simulink model "task_3s"  (R2021a)
settings: Solver=VariableStepAuto  StartTime=0  StopTime=140  RelTol=1e-3
values from neighbouring files (symbols this model uses):
  a0 = 600    [task_2.m]    (also in task_3.m)
  a1 = 4e3    (= 4000)    [task_2.m]    (also in task_3.m)
  a2 = 7.2e3    (= 7200)    [task_2.m]    (also in task_3.m)
  A_line = pi*D_line^2/4    (= 0.502654824574)    [task_2.m]    (also in task_3.m)
  A_p = pi*D_p^2/4    (= 0.441786466911)    [task_2.m]    (also in task_3.m)
  A_tank = pi*D_tank^2/4    (= 28.2743338823)    [task_2.m]    (also in task_3.m)
  beta_3 = 78*pi/180    (= 1.36135681656)    [task_2.m]    (also in task_3.m)
  Cd = 0.9    [task_2.m]    (also in task_3.m)
  D_line = 0.8    [task_2.m]    (also in task_3.m)
  D_p = 0.75    [task_2.m]    (also in task_3.m)
  D_w = 3.5    [task_2.m]    (also in task_3.m)
  g = 9.81    [task_2.m]    (also in task_3.m)
  h0 = 10    [task_2.m]    (also in task_3.m)
  h2 = 175    [task_2.m]    (also in task_3.m)
  h_tank_0 = 7.47    [task_2.m]    (also in task_3.m)
  J = 4.6e5    (= 460000)    [task_2.m]    (also in task_3.m)
  K = 2e9    (= 2000000000)    [task_2.m]    (also in task_3.m)
  L_line = 5    [task_2.m]    (also in task_3.m)
  L_p = 220    [task_2.m]    (also in task_3.m)
  lambda = 5e-3    (= 0.005)    [task_2.m]    (also in task_3.m)
  lambda_p = 1e-4    (= 0.0001)    [task_2.m]    (also in task_3.m)
  omega_t = 15    [task_2.m]    (also in task_3.m)
  p_amb = 1e5    (= 100000)    [task_2.m]    (also in task_3.m)
  psi = 0.97    [task_2.m]    (also in task_3.m)
  rho = 1000    [task_2.m]    (also in task_3.m)
  Rv = (Av0/pi)^(1/2)    (= 0.398942280401)    [task_2.m]    (also in task_3.m)
  V_c = 0.27    [task_2.m]    (also in task_3.m)
  V_p = A_p*L_p    (= 97.1930227204)    [task_2.m]    (also in task_3.m)
  x_v = 0.5    [task_2.m]    (also in task_3.m)
undefined symbols (not defined in the file or in its folder): magnitude
settings Model: Creator=Jihai  LastModifiedBy=Shinya
settings SolverCC: AlgebraicLoopSolver=TrustRegion
settings OptimizationCC: BlockReduction=off  DefaultParameterBehavior=Inlined  BufferReuse=off
settings DebuggingCC: SFMachineParentedDataDiag=warning

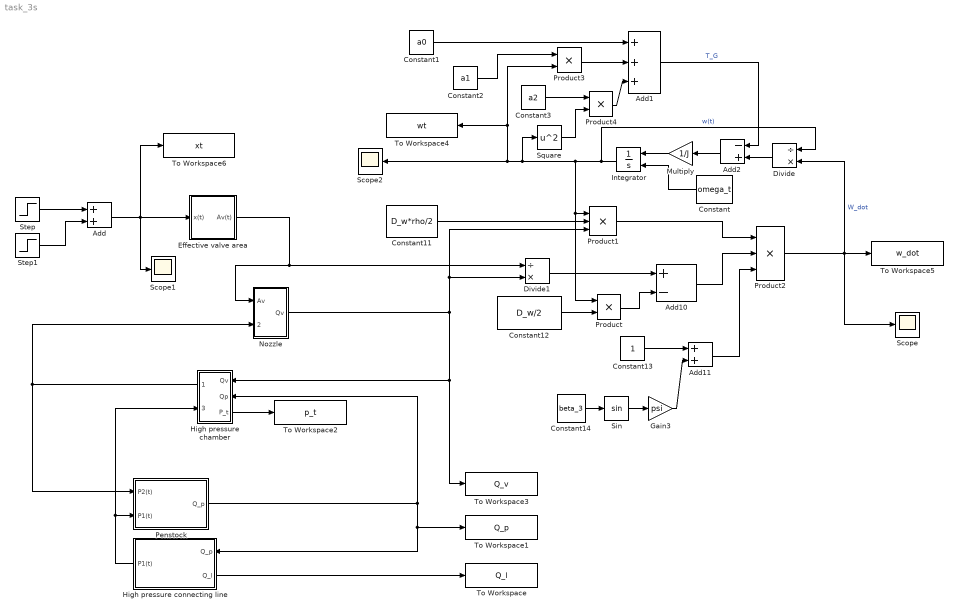
== system task_3s ==
  Add : Sum
  Add1 : Sum  Inputs=+++
  Add10 : Sum  Inputs=+-
  Add11 : Sum
  Add2 : Sum  Inputs=-+
  Constant : Constant  Value=omega_t
  Constant1 : Constant  Value=a0
  Constant11 : Constant  Value=D_w*rho/2
  Constant12 : Constant  Value=D_w/2
  Constant13 : Constant
  Constant14 : Constant  Value=beta_3
  Constant2 : Constant  Value=a1
  Constant3 : Constant  Value=a2
  Divide : Product  Inputs=/*
  Divide1 : Product  Inputs=/*
  Effective valve area : Subsystem
  Gain3 : Gain  Gain=psi
  High pressure chamber : Subsystem
      settings: PortSchema="{\"entries\":[{\"content\":{\"sides\":[{\"content\":{\"connectorIds\":[\"In1\",\"In2\",\"Out2\"]},\"type\":\"ConnectorPlacement.EquallySpacedRectSide\",\"uuid\":\"294ea827-fdb7-421d-abcf-acc1f7a75503\"},{\"content\":{\"connectorIds\":[\"Out1\",\"In3\"],\"side\":\"RIGHT\"},\"type\":\"ConnectorPlacement.EquallySpacedRectSide\",\"uuid\":\"1a834a5b-f580-4f55-8c0d-9c69e06391e8\"},{\"content\":{\"connectorIds\":[],\"side\":\"TOP\"},\"type\":\"ConnectorPlacement.EquallySpacedRectSide\",\"uuid\":\"b81bcc01-80a0-4387-ac31-2fde5e1e9cb3\"}]},\"type\":\"ConnectorPlacement.EquallySpacedConnector\",\"uuid\":\"9662d0fd-ac37-41a3-b53f-5a17ebe7bc5c\"}],\"packageUris\":[\"http://schema.mathworks.com/mf0/Connector/R2020b\"],\"version\":\"1.0\"}"
  High pressure connecting line : Subsystem
      settings: PortSchema="{\"entries\":[{\"content\":{\"sides\":[{\"content\":{\"connectorIds\":[\"In1\",\"Out2\"]},\"type\":\"ConnectorPlacement.EquallySpacedRectSide\",\"uuid\":\"6ad556de-4b40-4685-9767-8ac44a5f7b94\"},{\"content\":{\"connectorIds\":[\"Out1\"],\"side\":\"RIGHT\"},\"type\":\"ConnectorPlacement.EquallySpacedRectSide\",\"uuid\":\"0688f997-fb3f-4a41-bc89-421b9c81a19d\"},{\"content\":{\"connectorIds\":[],\"side\":\"TOP\"},\"type\":\"ConnectorPlacement.EquallySpacedRectSide\",\"uuid\":\"6829f08e-af19-4bca-bd06-6859c9ab2125\"}]},\"type\":\"ConnectorPlacement.EquallySpacedConnector\",\"uuid\":\"be56aa87-e3b2-4709-bfeb-a635322ac678\"}],\"packageUris\":[\"http://schema.mathworks.com/mf0/Connector/R2020b\"],\"version\":\"1.0\"}"
  Integrator : Integrator  InitialConditionSource=external
  Multiply : Gain  Gain=1/J
  Nozzle : Subsystem
  Penstock : Subsystem
  Product : Product
  Product1 : Product  Inputs=3
  Product2 : Product  Inputs=3
  Product3 : Product
  Product4 : Product
  Scope : Scope
  Scope1 : Scope
  Scope2 : Scope
  Sin : Trigonometry
  Square : Math  Operator=square  SaturateOnIntegerOverflow=on
  Step : Step  Time=20  Before=x_v  After=0.8  SampleTime=0
  Step1 : Step  Time=100  After=-0.7  SampleTime=0
  To Workspace : ToWorkspace  VariableName=Q_l  SampleTime=-1
  To Workspace1 : ToWorkspace  VariableName=Q_p  SampleTime=-1
  To Workspace2 : ToWorkspace  VariableName=p_t  SampleTime=-1
  To Workspace3 : ToWorkspace  VariableName=Q_v  SampleTime=-1
  To Workspace4 : ToWorkspace  VariableName=wt  SaveFormat=Timeseries  SampleTime=-1
  To Workspace5 : ToWorkspace  VariableName=w_dot  SaveFormat=Timeseries  SampleTime=-1
  To Workspace6 : ToWorkspace  VariableName=xt  SaveFormat=Timeseries  SampleTime=-1
  wires:
  High pressure chamber/1(P2(t)) -> Penstock/1(P2(t)), Nozzle/2(P2(t))
  Constant11/1 -> Product1/2
  Divide1/1 -> Add10/1
  Product1/1 -> Product2/1
  Add10/1 -> Product2/2
  Constant13/1 -> Add11/1
  Constant14/1 -> Sin/1
  Sin/1 -> Gain3/1
  Gain3/1 -> Add11/2
  Add11/1 -> Product2/3
  Product2/1 -> Divide/2, To Workspace5/1, Scope/1  "W_dot"
  High pressure connecting line/1(P1(t)) -> High pressure chamber/3(P1(t)), Penstock/2(P1(t))
  High pressure connecting line/2(Q_l) -> To Workspace/1
  Penstock/1(Q_p) -> High pressure chamber/2(Qp), High pressure connecting line/1(Q_p), To Workspace1/1
  Effective valve area/1(Av(t)) -> Nozzle/1(Av), Divide1/1
  High pressure chamber/2(P_t) -> To Workspace2/1
  Add/1 -> Scope1/1, To Workspace6/1, Effective valve area/1(x(t))
  Step/1 -> Add/1
  Step1/1 -> Add/2
  Nozzle/1(Qv) -> Product1/3, Divide1/2, To Workspace3/1, High pressure chamber/1(Qv)
  Constant/1 -> Integrator/2
  Product/1 -> Add10/2
  Constant12/1 -> Product/2
  Integrator/1 -> Divide/1, Square/1, To Workspace4/1, Product3/2, Scope2/1, Product1/1, Product/1  "w(t)"
  Divide/1 -> Add2/2
  Add1/1 -> Add2/1  "T_G"
  Add2/1 -> Multiply/1
  Multiply/1 -> Integrator/1
  Constant1/1 -> Add1/1
  Constant2/1 -> Product3/1
  Product4/1 -> Add1/3
  Product3/1 -> Add1/2
  Constant3/1 -> Product4/1
  Square/1 -> Product4/2

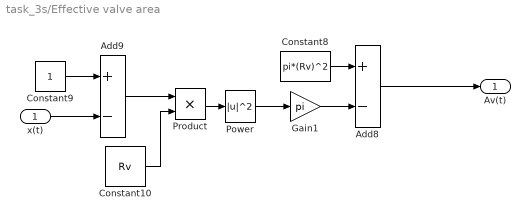
== system task_3s/Effective valve area ==
  x(t) : Inport
  Add8 : Sum  Inputs=+-
  Add9 : Sum  Inputs=+-
  Constant10 : Constant  Value=Rv
  Constant8 : Constant  Value=pi*(Rv)^2
  Constant9 : Constant
  Gain1 : Gain  Gain=pi
  Power : Math  Operator=magnitude^2  SaturateOnIntegerOverflow=on
  Product : Product
  Av(t) : Outport
  wires:
  Constant8/1 -> Add8/1
  Constant10/1 -> Product/2
  Add8/1 -> Av(t)/1
  Constant9/1 -> Add9/1
  Gain1/1 -> Add8/2
  Add9/1 -> Product/1
  Product/1 -> Power/1
  Power/1 -> Gain1/1
  x(t)/1 -> Add9/2

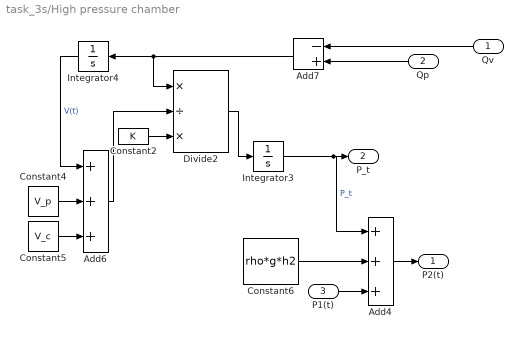
== system task_3s/High pressure chamber ==
  Qv : Inport
  Qp : Inport  Port=2
  P1(t) : Inport  Port=3
  Add4 : Sum  Inputs=+++
  Add6 : Sum  Inputs=+++
  Add7 : Sum  Inputs=-+
  Constant2 : Constant  Value=K
  Constant4 : Constant  Value=V_p
  Constant5 : Constant  Value=V_c
  Constant6 : Constant  Value=rho*g*h2
  Divide2 : Product  Inputs=*/*
  Integrator3 : Integrator
  Integrator4 : Integrator
  P2(t) : Outport
  P_t : Outport  Port=2
  wires:
  Add6/1 -> Divide2/2
  Add7/1 -> Divide2/1, Integrator4/1
  Integrator3/1 -> Add4/1, P_t/1  "P_t"
  Divide2/1 -> Integrator3/1
  Integrator4/1 -> Add6/1  "V(t)"
  Constant5/1 -> Add6/3
  Constant4/1 -> Add6/2
  Constant2/1 -> Divide2/3
  Qp/1 -> Add7/2
  Qv/1 -> Add7/1
  Constant6/1 -> Add4/2
  P1(t)/1 -> Add4/3
  Add4/1 -> P2(t)/1

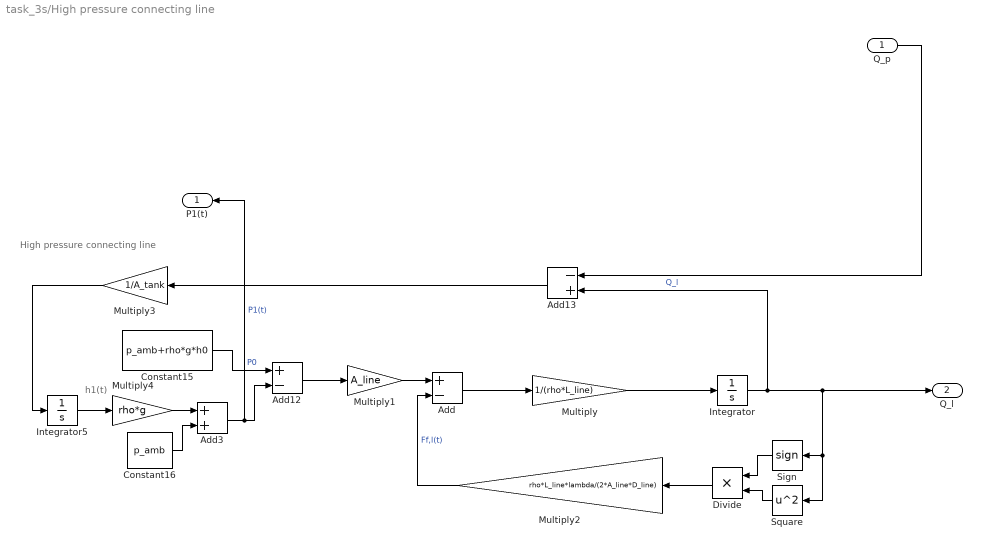
== system task_3s/High pressure connecting line ==
  note: High pressure connecting line
  note: h1(t)
  Q_p : Inport
  Add : Sum  Inputs=+-
  Add12 : Sum  Inputs=+-
  Add13 : Sum  Inputs=-+
  Add3 : Sum
  Constant15 : Constant  Value=p_amb+rho*g*h0
  Constant16 : Constant  Value=p_amb
  Divide : Product  Inputs=**
  Integrator : Integrator  InitialCondition=20
  Integrator5 : Integrator  InitialCondition=h_tank_0
  Multiply : Gain  Gain=1/(rho*L_line)
  Multiply1 : Gain  Gain=A_line
  Multiply2 : Gain  Gain=rho*L_line*lambda/(2*A_line*D_line)
  Multiply3 : Gain  Gain=1/A_tank
  Multiply4 : Gain  Gain=rho*g
  Sign : Signum
  Square : Math  Operator=square  SaturateOnIntegerOverflow=on
  P1(t) : Outport
  Q_l : Outport  Port=2
  wires:
  Integrator/1 -> Q_l/1, Sign/1, Square/1, Add13/2  "Q_l"
  Constant16/1 -> Add3/2
  Multiply4/1 -> Add3/1
  Q_p/1 -> Add13/1
  Multiply/1 -> Integrator/1
  Add/1 -> Multiply/1
  Constant15/1 -> Add12/1  "P0"
  Divide/1 -> Multiply2/1
  Add13/1 -> Multiply3/1
  Add12/1 -> Multiply1/1
  Multiply3/1 -> Integrator5/1
  Integrator5/1 -> Multiply4/1
  Multiply1/1 -> Add/1
  Add3/1 -> Add12/2, P1(t)/1  "P1(t)"
  Sign/1 -> Divide/1
  Square/1 -> Divide/2
  Multiply2/1 -> Add/2  "Ff,l(t)"

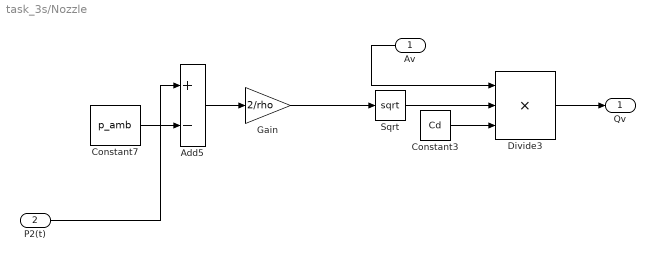
== system task_3s/Nozzle ==
  Av : Inport
  P2(t) : Inport  Port=2
  Add5 : Sum  Inputs=+-
  Constant3 : Constant  Value=Cd
  Constant7 : Constant  Value=p_amb
  Divide3 : Product  Inputs=***
  Gain : Gain  Gain=2/rho
  Sqrt : Sqrt  SaturateOnIntegerOverflow=on
  Qv : Outport
  wires:
  Constant7/1 -> Add5/2
  P2(t)/1 -> Add5/1
  Gain/1 -> Sqrt/1
  Sqrt/1 -> Divide3/2
  Constant3/1 -> Divide3/3
  Divide3/1 -> Qv/1
  Add5/1 -> Gain/1
  Av/1 -> Divide3/1

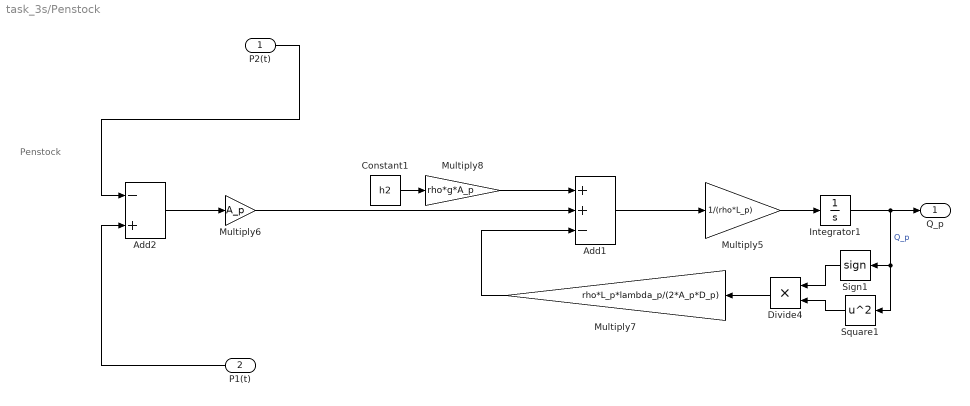
== system task_3s/Penstock ==
  note: Penstock
  P2(t) : Inport
  P1(t) : Inport  Port=2
  Add1 : Sum  Inputs=++-
  Add2 : Sum  Inputs=-+
  Constant1 : Constant  Value=h2
  Divide4 : Product  Inputs=**
  Integrator1 : Integrator  InitialCondition=20
  Multiply5 : Gain  Gain=1/(rho*L_p)
  Multiply6 : Gain  Gain=A_p
  Multiply7 : Gain  Gain=rho*L_p*lambda_p/(2*A_p*D_p)
  Multiply8 : Gain  Gain=rho*g*A_p
  Sign1 : Signum
  Square1 : Math  Operator=square  SaturateOnIntegerOverflow=on
  Q_p : Outport
  wires:
  Add2/1 -> Multiply6/1
  P1(t)/1 -> Add2/2
  Integrator1/1 -> Q_p/1, Square1/1, Sign1/1  "Q_p"
  Multiply7/1 -> Add1/3
  Divide4/1 -> Multiply7/1
  Add1/1 -> Multiply5/1
  Square1/1 -> Divide4/2
  Multiply5/1 -> Integrator1/1
  Sign1/1 -> Divide4/1
  Multiply8/1 -> Add1/1
  Multiply6/1 -> Add1/2
  Constant1/1 -> Multiply8/1
  P2(t)/1 -> Add2/1
